simulink model "vis_servo_DT_TR"  (R2020b)
settings: Solver=VariableStepAuto  StartTime=0.0  StopTime=100  RelTol=1e-3
values from neighbouring files (symbols this model uses):
  C_features_0 = homtrans(inv(W_T_C_0), W_features)    [init.m]
  C_features_desired = inv(O_T_C_desired) * O_features    [init.m]
  Cdesired_T_C0 = inv(C0_T_Cdesired)    [init.m]
  s_star_end = C_features_desired(:)    [init.m]
  Ts = 0.1    [init.m]    (also in test_for_c.m)
  W_T_C_0 = W_T_C_desired*SE3(R_0, t_0)    [init.m]
  W_T_C_desired = W_T_O*O_T_C_desired    [init.m]
undefined symbols (not defined in the file or in its folder): rotm2quat
libraries: simulink x1
settings Model: Creator=marco  LastModifiedBy=marco

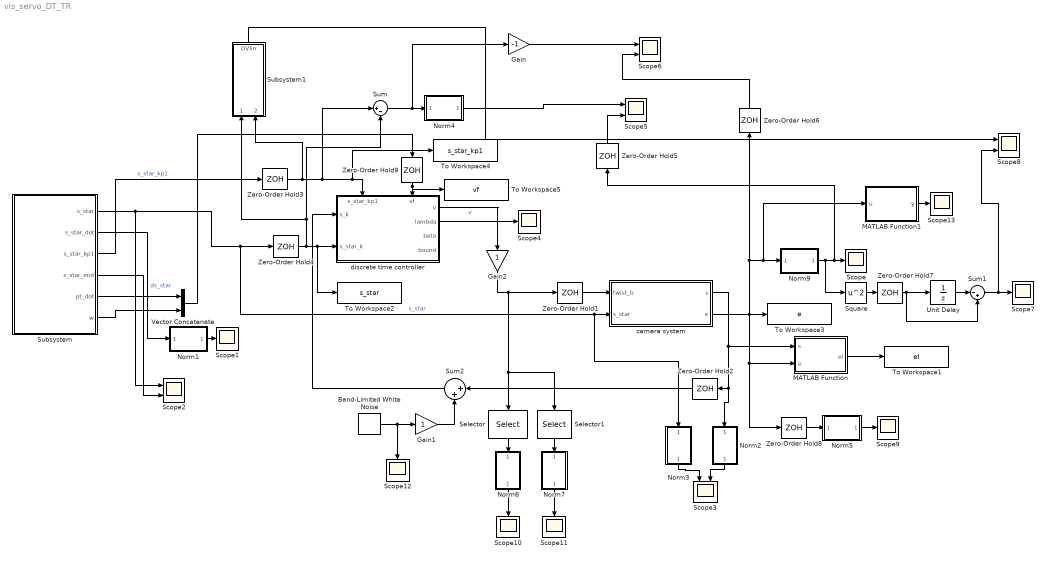
== system vis_servo_DT_TR ==
  Band-Limited White Noise : simulink/Sources/Band-Limited White Noise  Cov=[0.1]/1000^2/10 * ones([numel(C_features_desired),1])  Ts=Ts  seed=round(rand(numel(C_features_desired),1)*1000)
  Gain : Gain  Gain=-1
  Gain1 : Gain
  Gain2 : Gain
  MATLAB Function : MATLAB Function  TreatAsAtomicUnit=on
  MATLAB Function1 : MATLAB Function  TreatAsAtomicUnit=on
  Norm{1..7,9} (8 alike) : Subsystem  ReferencedSubsystem=Norm
  Scope{,1,4,7,9..13} (9 alike) : Scope
  Scope{2..3,5..6,8} (5 alike) : Scope  NumInputPorts=2
  Selector : Selector  InputPortWidth=6  IndexOptions=Index vector (dialog)  Indices=1:3  OutputSizes=1
  Selector1 : Selector  InputPortWidth=6  IndexOptions=Index vector (dialog)  Indices=4:6  OutputSizes=1
  Square : Math  Operator=square  SaturateOnIntegerOverflow=on
  Subsystem : Subsystem  mask{C_features_0=C_features_0, C_features_desired=C_features_desired, Cdesired_T_C0=Cdesired_T_C0.double, Ts=Ts, no_traj=on}
      mask prompts: C_features_0 "C_features_0 (initial features in camera frame)"; C_features_desired "C_features_desired (desired features in camera frame)"; Cdesired_T_C0 "Cdesired_T_C0 (camera initial frame w.r.t. camera desired frame)"
      mask Display:
      | disp('Ref Generator','texmode', 'on')
      | 
      | port_label('output',1,'s^*','texmode', 'on')
      | port_label('output',2,'ds^*','texmode', 'on')
      | port_label('output',3,'s^*_{k+1}','texmode', 'on')
      | port_label('output',4,'s^*_{END}','texmode', 'on')
      | port_label('output',5,'\dot{p_t}','texmode', 'on')
      | port_label('output',6,'\omega','texmode', 'on')
  Subsystem1 : Subsystem
  Sum : Sum  Inputs=|+-
  Sum1 : Sum  Inputs=|-+
  Sum2 : Sum  Inputs=|++
  To Workspace1 : ToWorkspace  VariableName=eI  SaveFormat=Timeseries  SampleTime=0.001
  To Workspace2 : ToWorkspace  VariableName=s_star  SaveFormat=Timeseries  SampleTime=-1
  To Workspace3 : ToWorkspace  VariableName=e  SaveFormat=Timeseries  SampleTime=0.001
  To Workspace4 : ToWorkspace  VariableName=s_star_kp1  SaveFormat=Timeseries  SampleTime=-1
  To Workspace5 : ToWorkspace  VariableName=vf  SaveFormat=Timeseries  SampleTime=-1
  Unit Delay : UnitDelay  InitialCondition=zeros(size(s_star_end))  SampleTime=Ts  HasFrameUpgradeWarning=on
  Vector Concatenate : Concatenate
  Zero-Order Hold{1..9} (9 alike) : ZeroOrderHold  SampleTime=Ts
  camera system : Subsystem  mask{W_p_C_0=W_T_C_0.t, W_q_C_0=rotm2quat(W_T_C_0.R)', s_star_end=s_star_end, W_T_Cd=W_T_C_desired.double}
  discrete time controller : Subsystem  mask{Ts=Ts, forward_action_enabled=off, vMax=0.2/2, wMax=0.5/3, use_majorant=off, use_lambda_const=off, lambdaT_const=0, use_max_analytic_lambda=off}
      settings: PortSchema="{\"entries\":[{\"content\":{\"sides\":[{\"content\":{\"connectorIds\":[\"In1\",\"In2\"]},\"type\":\"ConnectorPlacement.EquallySpacedRectSide\",\"uuid\":\"e89226d4-baa4-4c30-af13-ff098f2ce7fc\"},{\"content\":{\"connectorIds\":[\"Out1\",\"Out2\",\"Out3\",\"Out4\"],\"side\":\"RIGHT\"},\"type\":\"ConnectorPlacement.EquallySpacedRectSide\",\"uuid\":\"9d8bce32-3e74-4b83-8e79-37f4d5184f5a\"},{\"content\":{\"connectorIds\":[\"In3\",\"In4\"],\"side\":\"TOP\"},\"type\":\"ConnectorPlacement.EquallySpacedRectSide\",\"uuid\":\"9322580e-0316-476d-a1f3-db89d995a642\"},{\"content\":{\"connectorIds\":[],\"side\":\"HIDDEN\"},\"type\":\"ConnectorPlacement.EquallySpacedRectSide\",\"uuid\":\"a71e587c-d25e-434f-ae20-c6224730a5c7\"}]},\"type\":\"ConnectorPlacement.EquallySpacedConnector\",\"uuid\":\"c231d1ba-4204-4ba1-a9fd-ba17f6d657c2\"}],\"packageUris\":[\"http://schema.mathworks.com/mf0/Connector/R2020b\"],\"version\":\"1.0\"}"
      mask Display:
      | disp('Discrete Time Controller','texmode', 'on')
      | 
      | port_label('output',1,'v_k','texmode', 'on')
      | port_label('output',2,'\lambda_k','texmode', 'on')
      | port_label('output',3,'\beta_k','texmode', 'on')
      | port_label('output',4,'bound_k','texmode', 'on')
      | port_label('input',1,'s_k','texmode', 'on')
      | port_label('input',2,'s^*_k','texmode', 'on')
      | port_label('input',3,'s^*_{k+1}','texmode', 'on')
      | port_label('input',4,'vf','texmode', 'on')
  wires:
  Vector Concatenate/1 -> Zero-Order Hold9/1
  discrete time controller/1(v) -> Gain2/1  "v"
  camera system/1(s) -> MATLAB Function/1(s), Norm2/1, Zero-Order Hold2/1
  Sum2/1 -> discrete time controller/1(s_k)
  Subsystem/1(s_star) -> Scope2/1, Norm3/1, camera system/2(s_star), Zero-Order Hold4/1  "s_star"
  Subsystem/3(s_star_kp1) -> Zero-Order Hold3/1  "s_star_kp1"
  Zero-Order Hold3/1 -> Sum/1, To Workspace4/1, discrete time controller/3(s_star_kp1), Subsystem1/2(sstar_kp1)
  Zero-Order Hold4/1 -> To Workspace2/1, discrete time controller/2(s_star_k), Subsystem1/1(sstar_k), Sum/2
  camera system/2(e) -> Zero-Order Hold8/1, MATLAB Function/2(e), To Workspace3/1, MATLAB Function1/1(u), Norm9/1, Zero-Order Hold6/1
  MATLAB Function/1(eI) -> To Workspace1/1
  Norm1/1 -> Scope1/1
  Subsystem/2(s_star_dot) -> Norm1/1  "ds_star"
  Subsystem/4(s_star_end) -> Scope2/2
  Norm3/1 -> Scope3/1
  Norm2/1 -> Scope3/2
  discrete time controller/2(lambda) -> Scope4/1
  Sum/1 -> Gain/1, Norm4/1
  Norm4/1 -> Scope5/1
  Zero-Order Hold5/1 -> Scope5/2
  Gain/1 -> Scope6/1
  Zero-Order Hold6/1 -> Scope6/2
  Unit Delay/1 -> Sum1/1
  Sum1/1 -> Scope8/2, Scope7/1
  Norm9/1 -> Square/1, Zero-Order Hold5/1, Scope/1
  Zero-Order Hold7/1 -> Unit Delay/1, Sum1/2
  Square/1 -> Zero-Order Hold7/1
  Subsystem1/1(DVlin) -> Scope8/1
  Zero-Order Hold8/1 -> Norm5/1
  Norm5/1 -> Scope9/1
  Subsystem/5(pt_dot) -> Vector Concatenate/1
  Subsystem/6(w) -> Vector Concatenate/2
  Zero-Order Hold1/1 -> camera system/1(twist_b)
  Zero-Order Hold9/1 -> To Workspace5/1, discrete time controller/4(vf)
  Selector1/1 -> Norm7/1
  Selector/1 -> Norm6/1
  Norm6/1 -> Scope10/1
  Norm7/1 -> Scope11/1
  Zero-Order Hold2/1 -> Sum2/1
  Band-Limited White Noise/1 -> Gain1/1, Scope12/1
  Gain1/1 -> Sum2/2
  Gain2/1 -> Zero-Order Hold1/1, Selector1/1, Selector/1
  MATLAB Function1/1(y) -> Scope13/1

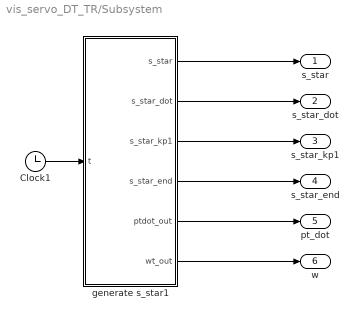
== system vis_servo_DT_TR/Subsystem ==
  Clock1 : Clock
  generate s_star1 : MATLAB Function  TreatAsAtomicUnit=on
  s_star : Outport
  s_star_dot : Outport  Port=2
  s_star_kp1 : Outport  Port=3
  s_star_end : Outport  Port=4
  pt_dot : Outport  Port=5
  w : Outport  Port=6
  wires:
  Clock1/1 -> generate s_star1/1(t)
  generate s_star1/3(s_star_kp1) -> s_star_kp1/1
  generate s_star1/1(s_star) -> s_star/1
  generate s_star1/2(s_star_dot) -> s_star_dot/1
  generate s_star1/4(s_star_end) -> s_star_end/1
  generate s_star1/5(ptdot_out) -> pt_dot/1
  generate s_star1/6(wt_out) -> w/1

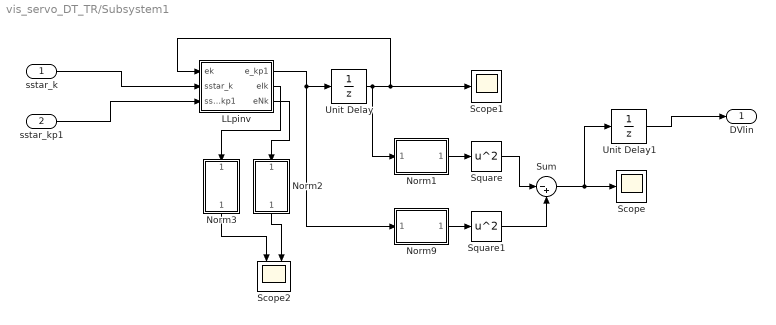
== system vis_servo_DT_TR/Subsystem1 ==
  sstar_k : Inport
  sstar_kp1 : Inport  Port=2
  LLpinv : MATLAB Function  TreatAsAtomicUnit=on
  Norm{1..3,9} (4 alike) : Subsystem  ReferencedSubsystem=Norm
  Scope : Scope
  Scope1 : Scope
  Scope2 : Scope  NumInputPorts=2
  Square : Math  Operator=square  SaturateOnIntegerOverflow=on
  Square1 : Math  Operator=square  SaturateOnIntegerOverflow=on
  Sum : Sum  Inputs=|-+
  Unit Delay : UnitDelay  InitialCondition=zeros(size(s_star_end))  SampleTime=-1  HasFrameUpgradeWarning=on
  Unit Delay1 : UnitDelay  InitialCondition=zeros(size(s_star_end))  SampleTime=-1  HasFrameUpgradeWarning=on
  DVlin : Outport
  wires:
  sstar_k/1 -> LLpinv/2(sstar_k)
  LLpinv/1(e_kp1) -> Norm9/1, Unit Delay/1
  sstar_kp1/1 -> LLpinv/3(sstar_kp1)
  Unit Delay/1 -> Norm1/1, Scope1/1, LLpinv/1(ek)
  Norm1/1 -> Square/1
  Norm9/1 -> Square1/1
  Square/1 -> Sum/1
  Square1/1 -> Sum/2
  Sum/1 -> Unit Delay1/1, Scope/1
  Unit Delay1/1 -> DVlin/1
  LLpinv/3(eNk) -> Norm2/1
  Norm2/1 -> Scope2/2
  LLpinv/2(eIk) -> Norm3/1
  Norm3/1 -> Scope2/1

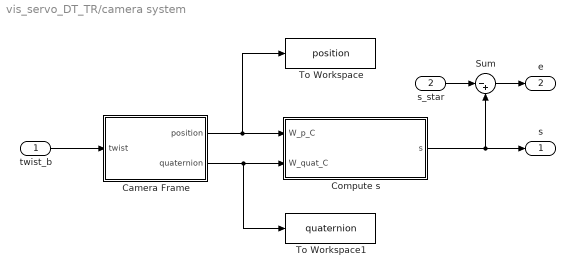
== system vis_servo_DT_TR/camera system ==
  twist_b : Inport
  s_star : Inport  Port=2
  Camera Frame : Subsystem
  Compute s : MATLAB Function  TreatAsAtomicUnit=on
  Sum : Sum  Inputs=|-+
  To Workspace : ToWorkspace  VariableName=position  SaveFormat=Timeseries  SampleTime=0.001
  To Workspace1 : ToWorkspace  VariableName=quaternion  SaveFormat=Timeseries  SampleTime=0.001
  s : Outport
  e : Outport  Port=2
  wires:
  Camera Frame/1(position) -> To Workspace/1, Compute s/1(W_p_C)
  Camera Frame/2(quaternion) -> To Workspace1/1, Compute s/2(W_quat_C)
  twist_b/1 -> Camera Frame/1(twist)
  Compute s/1(s) -> Sum/2, s/1
  Sum/1 -> e/1
  s_star/1 -> Sum/1

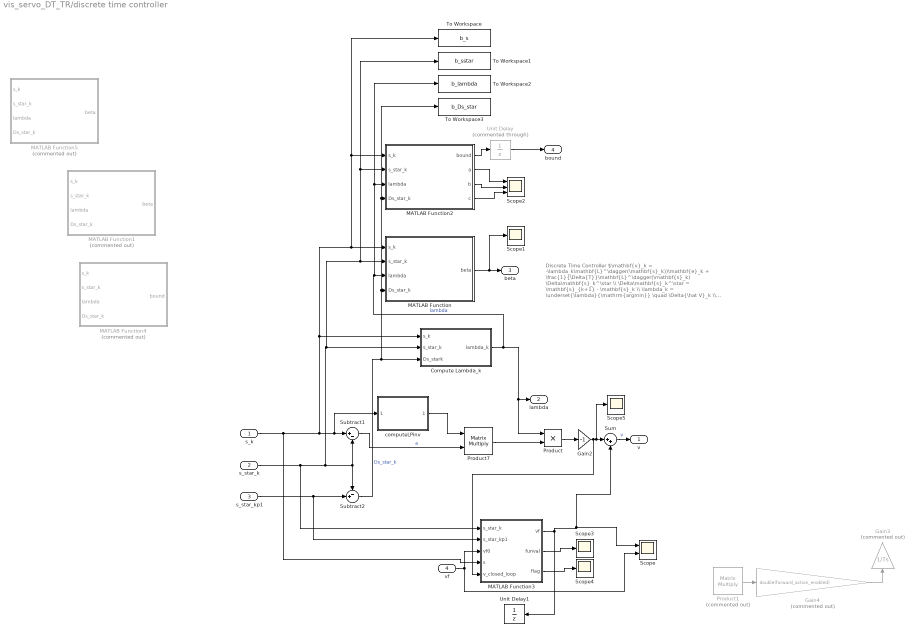
== system vis_servo_DT_TR/discrete time controller ==
  note: Discrete Time Controller
      | $\mathbf{v}_k = -\lambda_k\mathbf{L}^\dagger(\mathbf{s}_k))\mathbf{e}_k + \frac{1}{\Delta{T}}\mathbf{L}^\dagger(\mathbf{s}_k) \Delta\mathbf{s}_k^\star \\ \Delta\mathbf{s}_k^\star = \mathbf{s}_{k+1} - \mathbf{s}_k \\ \lambda_k = \underset{\lambda}{\mathrm{argmin}} \quad \Delta{\hat V}_k \\ \textrm{s.t.} \quad \textrm{velocity limits}$
  s_k : Inport
  s_star_k : Inport  Port=2
  s_star_kp1 : Inport  Port=3
  vf : Inport  Port=4
  Compute Lambda_k : Subsystem
  Gain2 : Gain  Gain=-1
  Gain3 : Gain  Commented=on  Gain=1/Ts
  Gain4 : Gain  Commented=on  Gain=double(forward_action_enabled)
  MATLAB Function : MATLAB Function  TreatAsAtomicUnit=on
  MATLAB Function1 : MATLAB Function  Commented=on  TreatAsAtomicUnit=on
  MATLAB Function2 : MATLAB Function  TreatAsAtomicUnit=on
  MATLAB Function3 : MATLAB Function  TreatAsAtomicUnit=on
  MATLAB Function4 : MATLAB Function  Commented=on  TreatAsAtomicUnit=on
  MATLAB Function5 : MATLAB Function  Commented=on  TreatAsAtomicUnit=on
  Product : Product
  Product1 : Product  Commented=on  Multiplication=Matrix(*)
  Product7 : Product  Multiplication=Matrix(*)
  Scope : Scope  NumInputPorts=2
  Scope{1,3..5} (4 alike) : Scope
  Scope2 : Scope  NumInputPorts=3
  Subtract1 : Sum  Inputs=|+-
  Subtract2 : Sum  Inputs=-+|
  Sum : Sum  Inputs=|++
  To Workspace : ToWorkspace  VariableName=b_s  SaveFormat=Timeseries  SampleTime=-1
  To Workspace1 : ToWorkspace  VariableName=b_sstar  SaveFormat=Timeseries  SampleTime=-1
  To Workspace2 : ToWorkspace  VariableName=b_lambda  SaveFormat=Timeseries  SampleTime=-1
  To Workspace3 : ToWorkspace  VariableName=b_Ds_star  SaveFormat=Timeseries  SampleTime=-1
  Unit Delay : UnitDelay  Commented=through  SampleTime=Ts  HasFrameUpgradeWarning=on
  Unit Delay1 : UnitDelay  InitialCondition=[0 0 0 0 0 0]'  SampleTime=Ts  HasFrameUpgradeWarning=on
  computeLPinv : Subsystem  ReferencedSubsystem=computeLPinv
  v : Outport
  lambda : Outport  Port=2
  beta : Outport  Port=3
  bound : Outport  Port=4
  wires:
  Subtract2/1 -> To Workspace3/1, MATLAB Function2/4(Ds_star_k), MATLAB Function/4(Ds_star_k), Compute Lambda_k/3(Ds_stark)  "Ds_star_k"
  Subtract1/1 -> Product7/2  "e"
  s_star_k/1 -> MATLAB Function3/1(s_star_k), To Workspace1/1, MATLAB Function2/2(s_star_k), MATLAB Function/2(s_star_k), Compute Lambda_k/2(s_star_k), Subtract2/1, Subtract1/2
  s_k/1 -> MATLAB Function3/4(s), To Workspace/1, MATLAB Function2/1(s_k), MATLAB Function/1(s_k), Compute Lambda_k/1(s_k), computeLPinv/1, Subtract1/1
  Compute Lambda_k/1(lambda_k) -> To Workspace2/1, MATLAB Function2/3(lambda), MATLAB Function/3(lambda), lambda/1, Product/1  "lambda"
  Product/1 -> Gain2/1
  Gain2/1 -> MATLAB Function3/5(v_closed_loop), Scope5/1, Sum/1
  Product7/1 -> Product/2
  Sum/1 -> v/1  "v"
  s_star_kp1/1 -> MATLAB Function3/2(s_star_kp1), Subtract2/2
  computeLPinv/1 -> Product7/1
  MATLAB Function/1(beta) -> Scope1/1, beta/1
  MATLAB Function2/1(bound) -> Unit Delay/1
  Unit Delay/1 -> bound/1
  MATLAB Function2/3(b) -> Scope2/2
  MATLAB Function2/2(a) -> Scope2/1
  MATLAB Function2/4(c) -> Scope2/3
  Gain4/1 -> Gain3/1
  Product1/1 -> Gain4/1
  MATLAB Function3/2(funval) -> Scope3/1
  MATLAB Function3/3(flag) -> Scope4/1
  MATLAB Function3/1(vf) -> Scope/1, Sum/2, Unit Delay1/1
  vf/1 -> MATLAB Function3/3(vf0), Scope/2

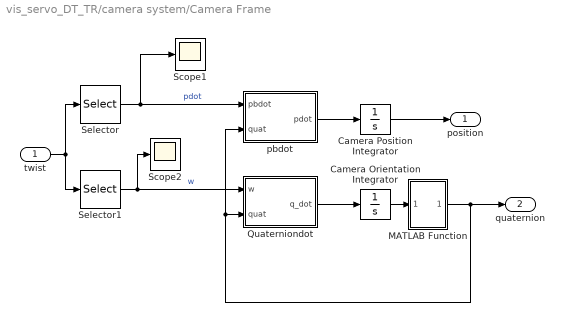
== system vis_servo_DT_TR/camera system/Camera Frame ==
  twist : Inport
  Camera Orientation Integrator : Integrator  InitialCondition=W_q_C_0
  Camera Position Integrator : Integrator  InitialCondition=W_p_C_0
  MATLAB Function : MATLAB Function  TreatAsAtomicUnit=on
  Quaterniondot : MATLAB Function  TreatAsAtomicUnit=on
  Scope1 : Scope
  Scope2 : Scope
  Selector : Selector  InputPortWidth=6  IndexOptions=Index vector (dialog)  Indices=[1:3]  OutputSizes=1
  Selector1 : Selector  InputPortWidth=6  IndexOptions=Index vector (dialog)  Indices=[4:6]  OutputSizes=1
  pbdot : MATLAB Function  TreatAsAtomicUnit=on
  position : Outport
  quaternion : Outport  Port=2
  wires:
  twist/1 -> Selector/1, Selector1/1
  Selector/1 -> Scope1/1, pbdot/1(pbdot)  "pdot"
  Selector1/1 -> Scope2/1, Quaterniondot/1(w)  "w"
  Camera Position Integrator/1 -> position/1
  Quaterniondot/1(q_dot) -> Camera Orientation Integrator/1
  Camera Orientation Integrator/1 -> MATLAB Function/1("quat ")
  pbdot/1(pdot) -> Camera Position Integrator/1
  MATLAB Function/1(quat) -> quaternion/1, pbdot/2(quat), Quaterniondot/2(quat)

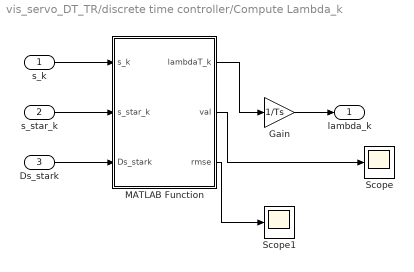
== system vis_servo_DT_TR/discrete time controller/Compute Lambda_k ==
  s_k : Inport
  s_star_k : Inport  Port=2
  Ds_stark : Inport  Port=3
  Gain : Gain  Gain=1/Ts
  MATLAB Function : MATLAB Function  TreatAsAtomicUnit=on
  Scope : Scope
  Scope1 : Scope
  lambda_k : Outport
  wires:
  s_k/1 -> MATLAB Function/1(s_k)
  s_star_k/1 -> MATLAB Function/2(s_star_k)
  Ds_stark/1 -> MATLAB Function/3(Ds_stark)
  MATLAB Function/1(lambdaT_k) -> Gain/1
  Gain/1 -> lambda_k/1
  MATLAB Function/2(val) -> Scope/1
  MATLAB Function/3(rmse) -> Scope1/1

== matlab function vis_servo_DT_TR/discrete time controller/MATLAB Function2 ==
  data: s_k input; bound output; a output; s_star_k input; lambda input; Ds_star_k input; Ts parameter; b output; c output
function [bound,a,b,c] = computeBound(s_k,s_star_k, lambda, Ds_star_k, Ts)

% bound = (1+lambda*Ts)/(lambda*Ts);b=0;return;

e = s_k-s_star_k;

L = computeL(s_k);
Lpinv = pinv(L);
eI = L*Lpinv*e;
eN = e - eI;

DsstarI = L*Lpinv*Ds_star_k;
DsstarN = Ds_star_k - DsstarI;

lT = lambda*Ts;
nEI = norm(eI);
nEN = norm(eN);
nE = norm(e);

nW1 = norm([zeros(3) eye(3)]*Lpinv*e);
if(nE < 10*eps)
    alpha = 1;
else
    alpha = (norm(e)/norm(eI));
end

% a = -lT;
% b = 2*abs(lT-1)+2;
% c = 1;

% a = -lT;
% b = 2/3+2*sqrt(abs(alpha^2-1))+1/(4*alpha);
% c = 1;

a = -lT;
b = 2*abs(lT-1)+2*sqrt(abs(alpha^2-1))+1/(4*alpha);
c = 1;

% a = -lT;
% b = 2+2*sqrt(abs(alpha^2-1))+1/(4*alpha);
% c = 1;

% a = -lT*(2-lT*(1+nW1*alpha));
% b = 2*abs(lT-1)+2*sqrt(abs(alpha^2-1))+lT^2*nW1;
% c = 1;

% bound = norm(Ds_star_k)* max(real(roots([a b c])));
bound = 0.03170* max(real(roots([a b c])));

return;

if false
   
    beta_vect = 0:0.001:100;
    pp = polyval([a b c], beta_vect);
    figure(100)
    plot(beta_vect,pp)
    grid on
    figure(99)
    plot(beta_vect,pp*norm(eI))
    grid on
    drawnow
    
end

== matlab function vis_servo_DT_TR/discrete time controller/MATLAB Function4 ==
  data: s_k input; bound output; s_star_k input; lambda input; Ds_star_k input; Ts parameter
function bound = computeBound(s_k,s_star_k, lambda, Ds_star_k, Ts)

Dsstar_max = 0.317;
use_dsstar_max = true;

alph_coeff = 1;

if norm(Ds_star_k) < 10*eps
    if(use_dsstar_max)
        bound = Dsstar_max;
    else
        bound = 0;
    end
   return;
end

e = s_k - s_star_k;

if norm(e) < 10*eps
    if(use_dsstar_max)
        bound = Dsstar_max;
    else
        bound = norm(Ds_star_k);
    end
   return;
end

L = computeL(s_k);
Lpinv = pinv(L);
eI = L*Lpinv*e;
eN = e - eI;

DsstarI = L*Lpinv*Ds_star_k;
DsstarN = Ds_star_k - DsstarI;

if(use_dsstar_max)
    nDss = Dsstar_max;
    nDssI = Dsstar_max;
    nDssN = Dsstar_max;
else
    nDss = norm(Ds_star_k);
    nDssI = norm(DsstarI);
    nDssN = norm(DsstarN);

    nDssI = nDss;
    nDssN = nDss;
end

lT = lambda*Ts;
nEI = norm(eI);
nEN = norm(eN);
nE = norm(e);

nW1 = norm([zeros(3) eye(3)]*Lpinv*e);
if(nEI < 10*eps)
    alph_w = 1 * alph_coeff;
else
    alph_w = ((nE + nDss)/nEI) * alph_coeff;
end
if(nE < 10*eps)
    alpha = 1 * alph_coeff;
else
    alpha = (norm(e)/norm(eI)) * alph_coeff;
end

a = -lT*(2-lT*(1+nW1*2*alph_w));
b = 2*(abs(lT-1)*nDssI+nDssN*2*alpha);
c = nDss^2;

bound = max(real(roots([a b c])));
return;

if false
   
    beta_vect = 0:0.001:100;
    pp = polyval([a b c], beta_vect);
    figure(100)
    plot(beta_vect,pp)
    grid on
    figure(99)
    plot(beta_vect,pp*norm(eI))
    grid on
    drawnow
    
end

== matlab function vis_servo_DT_TR/discrete time controller/MATLAB Function5 ==
  data: s_k input; beta output; s_star_k input; lambda input; Ds_star_k input; Ts parameter
function beta = computeBeta(s_k,s_star_k, lambda, Ds_star_k, Ts)

e = s_k - s_star_k;

L = computeL(s_k);
Lpinv = pinv(L);
eI = L*Lpinv*e;
eN = e - eI;

if(norm(e) < 10*eps)
    alpha = 1;
else
    alpha = norm(e)/norm(eI);
end


lT = lambda*Ts;
nEI = norm(eI);
nEN = norm(eN);
nE = norm(e);
nDss = norm(Ds_star_k);
nW1 = norm([zeros(3) eye(3)]*Lpinv*e);
a = -lT*(2-lT*(1+nW1*alpha));
b = 2*alpha^2*Ts*(1+lT);
c = alpha^2*Ts^2;

beta = max(real(roots([a b c])));
return;

if false
   
    beta_vect = 0:0.001:100;
    pp = polyval([a b c], beta_vect);
    figure(100)
    plot(beta_vect,pp)
    grid on
    figure(99)
    plot(beta_vect,pp*norm(eI))
    grid on
    drawnow
    
end

== matlab function vis_servo_DT_TR/Subsystem/generate s_star1 ==
  data: t input; s_star output; s_star_dot output; s_star_kp1 output; C_features_0 parameter double; s_star_end output; C_features_desired parameter double; Cdesired_T_C0 parameter double; Ts parameter double; no_traj parameter boolean; ptdot_out output; wt_out output
function [s_star,s_star_dot, s_star_kp1, s_star_end, ptdot_out,wt_out] = fcn(t, C_features_0, C_features_desired, Cdesired_T_C0, Ts, no_traj)

if no_traj
    s_star = C_features_desired(:);
    s_star_kp1 = C_features_desired(:);
    s_star_dot = zeros(size(s_star));
    s_star_end = C_features_desired(:);
    ptdot_out = zeros(3,1);
    wt_out = zeros(3,1);
    return
end

% common
pos_ti = 2*0;
ang_ti = 2*0;
useQuintic = true;
% trapz
MULT = .142 * 3 * 2.1;
pos_vmax = 0.05*2*3/3 *2 * 2 * 1.3 * MULT;
pos_ai = 0.5;
pos_af = 0.5;
w_max = deg2rad(10)/10*2*3/3 *2 * 2 * 1.3 * MULT;
ang_ai = deg2rad(10);
ang_af = deg2rad(10);
% quintic
pos_tf = pos_ti + (1/pos_vmax);
[~, ~, deltaAng] = quatInterp(t, [1 0 0 0], rotm2quat(Cdesired_T_C0(1:3,1:3)), @(t, deltaAng)trapezVelTraj(t,0,deltaAng,w_max,ang_ai,ang_af,ang_ti));
ang_tf = ang_ti + (deltaAng/w_max);

pos_tf = 2;
ang_tf = 2;

if useQuintic
    scalarTrajPos = @(t)quinticTraj(t,0,1,pos_ti,pos_tf);
    scalarTrajQuat = @(t,deltaAng)quinticTraj(t,0,deltaAng,ang_ti,ang_tf);
else
    scalarTrajPos = @(t)trapezVelTraj(t,0,1,pos_vmax,pos_ai,pos_af,pos_ti);
    scalarTrajQuat = @(t, deltaAng)trapezVelTraj(t,0,deltaAng,w_max,ang_ai,ang_af,ang_ti);
end

t_kp1 = t + Ts;

initial_quat = [1 0 0 0];
pi = [0;0;0];

final_quat = rotm2quat(Cdesired_T_C0(1:3,1:3));
pf = Cdesired_T_C0(1:3,4);

[Qt, wt] = quatInterp(t, initial_quat, final_quat, scalarTrajQuat);
Rt = quat2rotm(Qt);
[Qt_kp1] = quatInterp(t_kp1, initial_quat, final_quat, scalarTrajQuat);
Rt_kp1 = quat2rotm(Qt_kp1);
% Rt = Cdesired_T_C0(1:3,1:3);
% wt = [0 0 0]';

[pt, ptdot] = positionInterp(t, pi, pf, scalarTrajPos);
[pt_kp1] = positionInterp(t_kp1, pi, pf, scalarTrajPos);
% pt = Cdesired_T_C0(1:3,4);
% ptdot = [0 0 0]';

Tt = [Rt, pt; 0 0 0 1];
Tt_kp1 = [Rt_kp1, pt_kp1; 0 0 0 1];

FEATURE_star = homtrans(Tt, C_features_0);
FEATURE_star_kp1 = homtrans(Tt_kp1, C_features_0);
FEATURE_star_dot = zeros(size(FEATURE_star));
for i=1:size(C_features_0,2)
    FEATURE_star_dot(:,i) = skew(wt)*Rt*C_features_0(:,i) + ptdot(:);
%     FEATURE_star_dot(:,i) = Rt*skew(wt)*FEATURE_star(:,i) + ptdot(:);
end
wt_out = -wt;
ptdot_out = -(skew(pt)*wt + ptdot);
% wt_out = Rt*wt;
% ptdot_out = skew(pt)*Rt*wt + Rt*ptdot;
% wt_out = Rt'*wt;
% ptdot_out = -Rt'*skew(pt)*wt + Rt'*ptdot;

s_star = FEATURE_star(:);
s_star_kp1 = FEATURE_star_kp1(:);
s_star_dot = FEATURE_star_dot(:);
s_star_end = C_features_desired(:);

== matlab function vis_servo_DT_TR/camera system/Camera Frame/MATLAB Function ==
  data: quat input; quat output
function quat = fcn(quat)

quat = unit(quat);

== matlab function vis_servo_DT_TR/camera system/Camera Frame/Quaterniondot ==
  data: w input; q_dot output; quat input
function q_dot = fcn(w, quat)

q_dot = quat_dotb(quat,w);
% Q = UnitQuaternion(quat);
% Q_dot = Q.dot(w);
% q_dot = Q_dot.double'; 
% q_dot = [0 0 0 0]';

== matlab function vis_servo_DT_TR/camera system/Camera Frame/pbdot ==
  data: pbdot input; pdot output; quat input
function pdot = fcn(pbdot, quat)

W_R_B = quat2rotm(quat');
pdot = W_R_B*pbdot;

== matlab function vis_servo_DT_TR/camera system/Compute s ==
  data: W_p_C input; s output; W_quat_C input; s_star_end parameter; W_T_Cd parameter
function s = fcn(W_p_C, W_quat_C, s_star_end, W_T_Cd)

% W_T_C = SE3(quat2rotm(W_quat_C'),W_p_C);
W_T_C = [quat2rotm(W_quat_C'), W_p_C; 0 0 0 1];

% C_features = inv(W_T_C) * params.W_T_O * params.O_features;
C_T_Cd = invSE3(W_T_C) * W_T_Cd;
C_features = zeros(3,numel(s_star_end)/3);
C_features = homtrans(C_T_Cd, reshape(s_star_end,3,numel(s_star_end)/3));

s = C_features(:);

% s = params.O_features(:);

== matlab function vis_servo_DT_TR/MATLAB Function1 ==
  data: u input; y output
function y = fcn(u)

y = sqrt((norm(u)^2)/(numel(u)/3));

== matlab function vis_servo_DT_TR/MATLAB Function ==
  data: s input; eI output; e input
function eI = fcn(s, e)

L = computeL(s);
eI = L*pinv(L)*e;

== matlab function vis_servo_DT_TR/Subsystem1/LLpinv ==
  data: ek input; sstar_k input; e_kp1 output; eIk output; sstar_kp1 input; eNk output
function [e_kp1, eIk, eNk] = fcn(ek, sstar_k, sstar_kp1)

L = computeL(sstar_k);
Dsk = sstar_kp1 - sstar_k;

e_kp1 = (eye(numel(ek)) - L*pinv(L))*ek - Dsk;

eIk = L*pinv(L)*ek;
eNk = (eye(numel(ek)) - L*pinv(L))*ek;

== matlab function vis_servo_DT_TR/discrete time controller/MATLAB Function3 ==
  data: s_star_k input; vf output; s_star_kp1 input; vf0 input; s input; v_closed_loop input; Ts parameter; forward_action_enabled parameter; funval output; flag output
function [vf, funval, flag] = sim_forw_action(s_star_k,s_star_kp1, vf0, s, v_closed_loop,  Ts, forward_action_enabled)
    if forward_action_enabled
%         vf0 = zeros(6,1);
        [vf, funval, flag] = computeForwardAction(s_star_k, s_star_kp1, Ts, vf0, s, v_closed_loop(4:6));
    else
        vf0 = zeros(6,1);
        [vf, funval, flag] = computeForwardAction(s_star_k, s_star_k, Ts, vf0);
    end

== matlab function vis_servo_DT_TR/discrete time controller/MATLAB Function ==
  data: s_k input; beta output; s_star_k input; lambda input; Ds_star_k input; Ts parameter
function beta = computeBeta(s_k,s_star_k, lambda, Ds_star_k, Ts)

e = s_k - s_star_k;

L = computeL(s_k);
Lpinv = pinv(L);
eI = L*Lpinv*e;
eN = e - eI;

if(norm(e) < 10*eps)
    alpha = 1;
else
    alpha = norm(e)/norm(eI);
end


lT = lambda*Ts;
nEI = norm(eI);
nEN = norm(eN);
nE = norm(e);
nDss = norm(Ds_star_k);
nW1 = norm([zeros(3) eye(3)]*Lpinv*e);
% a = -lT*(2-lT*(1+nW1*alpha));
% b = 2*alpha^2*Ts*(1+lT);
% c = alpha^2*Ts^2;

% a = -lT*(2-lT*(1+nW1*alpha));
% b = 2*alpha*Ts*(alpha+lT);
% c = alpha^2*Ts^2;

% alpha = 1;
% nW1 = 0;
% lambda = 1/Ts;

% c = Ts^2*alpha^2;
% b = Ts*alpha*(2*abs(lambda*Ts-1) + 2*sqrt(alpha^2-1) + (lambda*Ts)^2*nW1 );
% a = -lambda*Ts*(2-alpha*lambda*Ts*nW1 - lambda*Ts);

c = Ts^2*alpha^2;
b = Ts*alpha*(2*abs(lambda*Ts-1) + 2*sqrt(abs(alpha^2-1)) + 1/(4*alpha) );
a = -lambda*Ts;

beta = max(real(roots([a b c])));

== matlab function vis_servo_DT_TR/discrete time controller/Compute Lambda_k/MATLAB Function ==
  data: s_k input; lambdaT_k output; s_star_k input; Ds_stark input; Ts parameter double; vMax parameter double; wMax parameter double; forward_action_enabled parameter boolean; use_majorant parameter boolean; use_lambda_const parameter boolean; lambdaT_const parameter double; use_max_analytic_lambda parameter boolean; val output; rmse output
function [lambdaT_k, val, rmse] = fcn(s_k, s_star_k, Ds_stark, Ts, vMax, wMax, forward_action_enabled, use_majorant, use_lambda_const, lambdaT_const, use_max_analytic_lambda)
coder.extrinsic('opt_problem_lambdaT'); % <- Informing the Coder

val = 0;
rmse = 0;

if use_lambda_const
    lambdaT_k = lambdaT_const;
    return;
end

ek = s_k-s_star_k;

if use_max_analytic_lambda
   lambdaT_k = computeAnaliticLambdaTMax(ek,computeL(s_k),Ds_stark)/2;
   return;
end


% lambdaT_k = opt_problem_lambdaT(...
%     ek,...
%     s_star_k,...
%     Ts,...
%     vMax,...
%     wMax,...
%     Ds_stark,...
%     forward_action_enabled,...
%     use_majorant...
%     );

lambdaT_k = opt_problem_lambdaT(...
    ek, ...
    s_star_k, ...
    vMax*Ts, ...
    wMax*Ts, ...
    Ds_stark, ...
    forward_action_enabled, ...
    use_majorant ...
    );

return
MIN = 0.002;
MAX = 0.005;
valMIN = Ts;
valMAX = 1;
rmse = sqrt(norm(ek)^2/(numel(ek)/3));
if rmse > MAX
    val = 1;
elseif rmse < MIN
    val = valMIN;
else
    val = (valMIN-valMAX)/(MIN-MAX) * rmse - (valMIN-valMAX)/(MIN-MAX) * MAX + valMAX;
end
lambdaT_k = lambdaT_k*val;

== matlab function vis_servo_DT_TR/discrete time controller/MATLAB Function1 ==
  data: s_k input; beta output; s_star_k input; lambda input; Ds_star_k input; Ts parameter
function beta = computeBeta(s_k,s_star_k, lambda, Ds_star_k, Ts)

e = s_k - s_star_k;

L = computeL(s_k);
Lpinv = pinv(L);
eI = L*Lpinv*e;
eN = e - eI;

if(norm(e) < 10*eps)
    alpha = 1;
else
    alpha = norm(e)/norm(eI);
    if 1-alpha < 1e-5
        alpha = 1;
    end
end
if(alpha < 1)
    dummy = 0;
end

vel1 = - Lpinv*e + Lpinv*Ds_star_k/(lambda*Ts);
% vel1 = - Lpinv*e;
omega1 = vel1(4:6);

% a = -2*lambda*Ts*(1-alpha*lambda*Ts*.5*norm(omega1)-.5*lambda*Ts);
% b = 2*alpha*(sqrt(alpha^2-1) + lambda*Ts*.5*norm(omega1)*(alpha+lambda*Ts*(1+lambda*Ts*.5*norm(omega1))));
% c = alpha^2*Ts*((1+lambda*Ts*.5*norm(omega1))^2);

% omega = [zeros(3) eye(3)]*Lpinv*(Ds_star_k/Ts - lambda*e);
% a = -2*lambda*Ts*(1-alpha*lambda*Ts*.5*norm([zeros(3) eye(3)]*Lpinv*e)-alpha*.5*norm([zeros(3) eye(3)]*Lpinv*Ds_star_k)-.5*lambda*Ts);
% b = 2*alpha*Ts*( sqrt(alpha^2-1) + .5*Ts*norm(omega)*(alpha + lambda*Ts*(1+.5*Ts*norm(omega))));
% c = alpha^2*Ts^2*(1+.5*Ts*norm(omega))^2;

% alpg t/2 *norm(omegakf)
% norm(omegakf) <= sigmamax([o I]Lpinv)*norm(Dsstark)/T <= sigmamax([o I]Lpinv)*sdotM <= sigmamax([o I]Lpinv)*norm(e)/beta
% alph T/2*sigmamax([o I]Lpinv)*norm(e)/beta
% ---
% lambdak*T*sigmamax([o I]Lpinv)*ek beta

% omega = [zeros(3) eye(3)]*Lpinv*(Ds_star_k/Ts - lambda*e);
% sigmamax = max(svd([zeros(3) eye(3)]*Lpinv));
% termine = lambda*Ts*sigmamax*norm(e);
% a = -2*lambda*Ts*(1-alpha*lambda*Ts*.5*norm([zeros(3) eye(3)]*Lpinv*e)-.5*lambda*Ts);
% b = termine + 2*alpha*Ts*( sqrt(alpha^2-1) + .5*Ts*norm(omega)*(alpha + lambda*Ts*(1+.5*Ts*norm(omega))));
% c = alpha^2*Ts^2*(1+.5*Ts*norm(omega))^2;

% lT = lambda*Ts;
% nEI = norm(eI);
% nEN = norm(eN);
% nE = norm(e);
% alph_e = alpha;
% nW1 = norm([zeros(3) eye(3)]*Lpinv*e);
% a = -lT*nEI^2*(2-lT*(1+nW1)*alph_e);
% b = 2*abs(lT-1)*nE*nEI+2*nE*nEN+lT^2*nW1*alph_e;
% c = nE^2;
% if nE < 1e-5
%    beta = nan;
%    return;
% end


lT = lambda*Ts;
nEI = norm(eI);
nEN = norm(eN);
nE = norm(e);
alph_e = alpha;
nDss = norm(Ds_star_k);
nW1 = norm([zeros(3) eye(3)]*Lpinv*e);
if(nEI < 10*eps)
    alph_w = 1;
else
    alph_w = (nE + norm(nDss))/nEI;
end
a = -lT*(2-lT*(1+nW1*alph_w));
b = 2*(abs(lT-1)*nDss+nDss*alph_e);
c = nDss^2;

beta = max(real(roots([a b c])));
return;

if false
   
    beta_vect = 0:0.001:100;
    pp = polyval([a b c], beta_vect);
    figure(100)
    plot(beta_vect,pp)
    grid on
    figure(99)
    plot(beta_vect,pp*norm(eI))
    grid on
    drawnow
    
end


DELTA = b^2 - 4*a*c;
if(DELTA < 0)
   beta = 0;
   return;
end
sol1 = (-b - sqrt(DELTA))/2*a;
sol2 = (-b + sqrt(DELTA))/2*a;

if sol1*sol2 <= 0
   beta = max(sol1,sol2); 
   return; % OK
end

if sol1 < 0
    beta = 0; % both negative impossible
    return;
end

% if sol1 > 0
   beta = max(sol1,sol2); % impossible
   return;
% end
